simulink model "ec_fixed_config_subsys"  (Simulink 10.0)
settings: Solver=FixedStepDiscrete  StartTime=0.0  StopTime=20  RelTol=1e-3
PreLoadFcn:
  | ec_fixed_setup;
StartFcn:
  | tic;
StopFcn:
  | toc;
undefined symbols (not defined in the file): Fs, pic_frame_size
libraries: dspsrcs4 x9, ec_lib x6, simulink x6
settings Model: Creator=Kerry Schutz  LastModifiedBy=bhisma
settings DataIOCC: LimitDataPoints=on  SignalLoggingSaveFormat=ModelDataLogs
settings OptimizationCC: DefaultParameterBehavior=Inlined  InlineInvariantSignals=on  ExpressionDepthLimit=2147483647  StateBitsets=on  DataBitsets=on  ZeroExternalMemoryAtStartup=off  ZeroInternalMemoryAtStartup=off  EfficientFloat2IntCast=on  LifeSpan=1  EfficientTunableParamExpr=on
settings DebuggingCC: AlgebraicLoopMsg=none  SaveWithParameterizedLinksMsg=none  SolverPrmCheckMsg=warning  FcnCallInpInsideContextMsg=warning  StateNameClashWarn=warning
settings HardwareCC: ProdBitPerInt=16  ProdBitPerPointer=16  ProdBitPerSizeT=16  ProdBitPerPtrDiffT=16  ProdIntDivRoundTo=Zero  ProdEndianess=LittleEndian  ProdWordSize=16  ProdHWDeviceType=Microchip->dsPIC  TargetHWDeviceType=32-bit Generic
settings SFSimCC: SimUseLocalCustomCode=on  SimParseCustomCode=off  MATLABDynamicMemAlloc=off  CustomCodeUndefinedFunction=FilterOut
settings RTWCC: Description=Real-Time Workshop Embedded Coder (no auto configuration)  SystemTargetFile=ert.tlc  GenCodeOnly=on  TemplateMakefile=ert_default_tmf  RTWUseLocalCustomCode=on  CreateSILPILBlock=SIL
settings CodeAppCC: IgnoreCustomStorageClasses=off  CustomSymbolStrType=$N$R$M  InternalIdentifier=Classic  InlinedPrmAccess=Macros
settings ERTTargetCC: TargetFcnLib=ansi_tfl_tmw.mat  GenerateSampleERTMain=on  IncludeMdlTerminateFcn=off  SupportAbsoluteTime=off  PurelyIntegerCode=on  SupportNonFinite=off  SupportComplex=off  InlinedParameterPlacement=NonHierarchical  ERTCustomFileTemplate=example_file_process.tlc  ConvertIfToSwitch=off  SuppressUnreachableDefaultCases=off

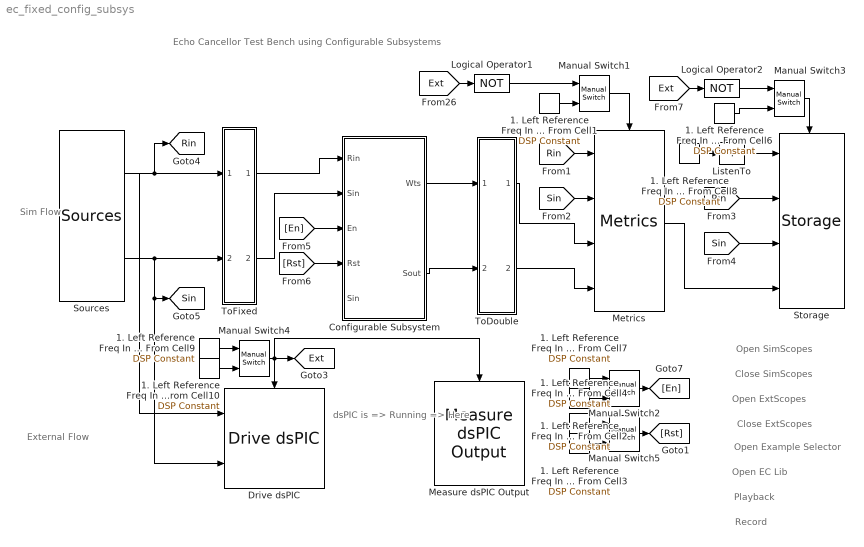
== system ec_fixed_config_subsys ==
  note: Echo Cancellor Test Bench using Configurable Subsystems
  note: Sim
      | Flow
  note: dsPIC is
      | => Running  =>
      |   Here
  note: External
      | Flow
  note: Playback
  note: Record
  note: Open EC Lib
  note: Open Example Selector
  note: Close SimScopes
  note: Open ExtScopes
  note: Close ExtScopes
  note: Open SimScopes
  1. Left Reference Freq In Hz From Cell1 : dspsrcs4/DSP Constant  SystemSampleTime=-1  Value=0  SampleMode=Discrete  discreteOutput=Sample-based  continuousOutput=Sample-based  sampTime=pic_frame_size/Fs  framePeriod=pic_frame_size/Fs  dataType=double  isSigned=on  wordLen=16  udDataType=sfix(16)  fracBitsMode=Best precision  numFracBits=15  InterpretAs1D=-inf  Ts=-inf  FramebasedOutput=-inf
      settings: SourceProductName=DSP System Toolbox  SourceProductBaseCode=DS  additionalParams=on
  1. Left Reference Freq In Hz From Cell10 : dspsrcs4/DSP Constant  SystemSampleTime=-1  Value=0  SampleMode=Discrete  discreteOutput=Sample-based  continuousOutput=Sample-based  sampTime=pic_frame_size/Fs  framePeriod=pic_frame_size/Fs  dataType=double  isSigned=on  wordLen=16  udDataType=sfix(16)  fracBitsMode=Best precision  numFracBits=15  InterpretAs1D=-inf  Ts=-inf  FramebasedOutput=-inf
      settings: SourceProductName=DSP System Toolbox  SourceProductBaseCode=DS  additionalParams=on
  1. Left Reference Freq In Hz From Cell2 : dspsrcs4/DSP Constant  SystemSampleTime=-1  Value=0  SampleMode=Discrete  discreteOutput=Sample-based  continuousOutput=Sample-based  sampTime=pic_frame_size/Fs  framePeriod=pic_frame_size/Fs  dataType=int16  isSigned=on  wordLen=16  udDataType=sfix(16)  fracBitsMode=Best precision  numFracBits=15  InterpretAs1D=-inf  Ts=-inf  FramebasedOutput=-inf
      settings: SourceProductName=DSP System Toolbox  SourceProductBaseCode=DS  additionalParams=on
  1. Left Reference Freq In Hz From Cell3 : dspsrcs4/DSP Constant  SystemSampleTime=-1  Value=0  SampleMode=Discrete  discreteOutput=Sample-based  continuousOutput=Sample-based  sampTime=pic_frame_size/Fs  framePeriod=pic_frame_size/Fs  dataType=int16  isSigned=on  wordLen=16  udDataType=sfix(16)  fracBitsMode=Best precision  numFracBits=15  InterpretAs1D=-inf  Ts=-inf  FramebasedOutput=-inf
      settings: SourceProductName=DSP System Toolbox  SourceProductBaseCode=DS  additionalParams=on
  1. Left Reference Freq In Hz From Cell4 : dspsrcs4/DSP Constant  SystemSampleTime=-1  Value=1  SampleMode=Discrete  discreteOutput=Sample-based  continuousOutput=Sample-based  sampTime=pic_frame_size/Fs  framePeriod=pic_frame_size/Fs  dataType=int16  isSigned=on  wordLen=16  udDataType=sfix(16)  fracBitsMode=Best precision  numFracBits=15  InterpretAs1D=-inf  Ts=-inf  FramebasedOutput=-inf
      settings: SourceProductName=DSP System Toolbox  SourceProductBaseCode=DS  additionalParams=on
  1. Left Reference Freq In Hz From Cell6 : dspsrcs4/DSP Constant  SystemSampleTime=-1  Value=0  SampleMode=Discrete  discreteOutput=Sample-based  continuousOutput=Sample-based  sampTime=pic_frame_size/Fs  framePeriod=2  dataType=double  isSigned=on  wordLen=16  udDataType=sfix(16)  fracBitsMode=Best precision  numFracBits=15  InterpretAs1D=-inf  Ts=-inf  FramebasedOutput=-inf
      settings: SourceProductName=DSP System Toolbox  SourceProductBaseCode=DS  additionalParams=on
  1. Left Reference Freq In Hz From Cell7 : dspsrcs4/DSP Constant  SystemSampleTime=-1  Value=1  SampleMode=Discrete  discreteOutput=Sample-based  continuousOutput=Sample-based  sampTime=pic_frame_size/Fs  framePeriod=pic_frame_size/Fs  dataType=int16  isSigned=on  wordLen=16  udDataType=sfix(16)  fracBitsMode=Best precision  numFracBits=15  InterpretAs1D=-inf  Ts=-inf  FramebasedOutput=-inf
      settings: SourceProductName=DSP System Toolbox  SourceProductBaseCode=DS  additionalParams=on
  1. Left Reference Freq In Hz From Cell8 : dspsrcs4/DSP Constant  SystemSampleTime=-1  Value=1  SampleMode=Discrete  discreteOutput=Sample-based  continuousOutput=Sample-based  sampTime=pic_frame_size/Fs  framePeriod=2  dataType=double  isSigned=on  wordLen=16  udDataType=sfix(16)  fracBitsMode=Best precision  numFracBits=15  InterpretAs1D=-inf  Ts=-inf  FramebasedOutput=-inf
      settings: SourceProductName=DSP System Toolbox  SourceProductBaseCode=DS  additionalParams=on
  1. Left Reference Freq In Hz From Cell9 : dspsrcs4/DSP Constant  SystemSampleTime=-1  Value=1  SampleMode=Discrete  discreteOutput=Sample-based  continuousOutput=Sample-based  sampTime=pic_frame_size/Fs  framePeriod=pic_frame_size/Fs  dataType=double  isSigned=on  wordLen=16  udDataType=sfix(16)  fracBitsMode=Best precision  numFracBits=15  InterpretAs1D=-inf  Ts=-inf  FramebasedOutput=-inf
      settings: SourceProductName=DSP System Toolbox  SourceProductBaseCode=DS  additionalParams=on
  Configurable Subsystem : Subsystem  BlockChoice=SLM16 codegen
      settings: AttributesFormatString=%<BlockChoice>  MemberBlocks=LCT sim,SLM16 codegen,SLM16 sim,SLP FORi,SLP Force
      settings: TemplateBlock=|
      | ec_lib/Configurable
      | Subsystem
  Drive dsPIC : ec_lib/Drive dsPIC  SystemSampleTime=-1
  ListenTo : simulink/Math Operations/Slider Gain  SystemSampleTime=-1  low=0  gain=4  high=10
  Logical Operator1 : Logic  Operator=NOT  AllPortsSameDT=off  OutDataTypeStr=boolean
  Logical Operator2 : Logic  Operator=NOT  AllPortsSameDT=off  OutDataTypeStr=boolean
  Manual Switch1 : simulink/Signal Routing/Manual Switch  SystemSampleTime=-1  sw=1  action=0  varsize=off
      settings: SourceProductName=Simulink  SourceProductBaseCode=SL
  Manual Switch2 : simulink/Signal Routing/Manual Switch  SystemSampleTime=-1  sw=1  action=0  varsize=off
      settings: SourceProductName=Simulink  SourceProductBaseCode=SL
  Manual Switch3 : simulink/Signal Routing/Manual Switch  SystemSampleTime=-1  sw=1  action=0  varsize=off
      settings: SourceProductName=Simulink  SourceProductBaseCode=SL
  Manual Switch4 : simulink/Signal Routing/Manual Switch  SystemSampleTime=-1  sw=0  action=0  varsize=off
      settings: SourceProductName=Simulink  SourceProductBaseCode=SL
  Manual Switch5 : simulink/Signal Routing/Manual Switch  SystemSampleTime=-1  sw=0  action=0  varsize=off
      settings: SourceProductName=Simulink  SourceProductBaseCode=SL
  Measure dsPIC Output : ec_lib/Measure dsPIC Output  SystemSampleTime=-1
  Metrics : ec_lib/Metrics  SystemSampleTime=-1
  Sources : ec_lib/Sources  SystemSampleTime=-1
  Storage : ec_lib/Storage  SystemSampleTime=-1
  ToDouble : Subsystem
  ToFixed : Subsystem
  tag scope: Ext=global, Rin=global, Sin=global
  wires:
  1. Left Reference Freq In Hz From Cell6/1 -> Manual Switch3/2
  Manual Switch3/1 -> Storage/Enable
  1. Left Reference Freq In Hz From Cell10/1 -> Manual Switch4/2
  1. Left Reference Freq In Hz From Cell9/1 -> Manual Switch4/1
  Manual Switch4/1 -> [Ext], Drive dsPIC/Enable, Measure dsPIC Output/Enable
  ListenTo/1 -> Storage/1
  1. Left Reference Freq In Hz From Cell8/1 -> ListenTo/1
  ToFixed/1(Rin) -> Configurable Subsystem/1(Rin)
  Configurable Subsystem/1(Wts) -> ToDouble/1(In1)
  Configurable Subsystem/2(Sout) -> ToDouble/2(In2)
  Sources/2 -> ToFixed/2(" In2"), [Sin], Drive dsPIC/2
  Sources/1 -> ToFixed/1(In1), [Rin], Drive dsPIC/1
  ToDouble/1(Wts) -> Metrics/3
  ToDouble/2(Sout) -> Metrics/4
  Metrics/1 -> Storage/4
  1. Left Reference Freq In Hz From Cell1/1 -> Manual Switch1/2
  Manual Switch1/1 -> Metrics/Enable
  [Ext] -> Logical Operator1/1
  [Rin] -> Metrics/1
  [Sin] -> Metrics/2
  [Rin] -> Storage/2
  [Sin] -> Storage/3
  1. Left Reference Freq In Hz From Cell7/1 -> Manual Switch2/1
  Manual Switch2/1 -> [En]
  1. Left Reference Freq In Hz From Cell2/1 -> Manual Switch2/2
  1. Left Reference Freq In Hz From Cell4/1 -> Manual Switch5/1
  Manual Switch5/1 -> [Rst]
  1. Left Reference Freq In Hz From Cell3/1 -> Manual Switch5/2
  [En] -> Configurable Subsystem/3(En)
  [Rst] -> Configurable Subsystem/4(Rst)
  Logical Operator1/1 -> Manual Switch1/1
  [Ext] -> Logical Operator2/1
  Logical Operator2/1 -> Manual Switch3/1
  ToFixed/2(Sin) -> Configurable Subsystem/2("Sin ")

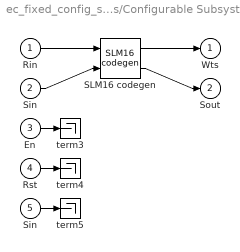
== system ec_fixed_config_subsys/Configurable Subsystem ==
  Rin : Inport
  "Sin " : Inport  Port=2
  En : Inport  Port=3
  Rst : Inport  Port=4
  Sin : Inport  Port=5
  SLM16 codegen : ec_lib/SLM16 codegen  SystemSampleTime=-1
  term3 : Terminator
  term4 : Terminator
  term5 : Terminator
  Wts : Outport
  Sout : Outport  Port=2
  wires:
  Rin/1 -> SLM16 codegen/1
  "Sin "/1 -> SLM16 codegen/2
  SLM16 codegen/1 -> Wts/1
  SLM16 codegen/2 -> Sout/1
  En/1 -> term3/1
  Rst/1 -> term4/1
  Sin/1 -> term5/1

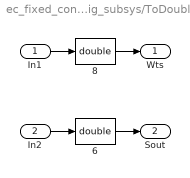
== system ec_fixed_config_subsys/ToDouble ==
  In1 : Inport
  In2 : Inport  Port=2
  " 6" : DataTypeConversion  OutDataTypeStr=double
  " 8" : DataTypeConversion  OutDataTypeStr=double
  Wts : Outport
  Sout : Outport  Port=2
  wires:
  In1/1 -> " 8"/1
  " 8"/1 -> Wts/1
  In2/1 -> " 6"/1
  " 6"/1 -> Sout/1

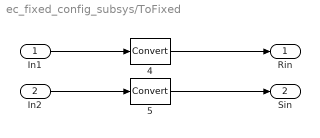
== system ec_fixed_config_subsys/ToFixed ==
  In1 : Inport
  " In2" : Inport  Port=2
  " 4" : DataTypeConversion
  " 5" : DataTypeConversion
  Rin : Outport
  Sin : Outport  Port=2
  wires:
  In1/1 -> " 4"/1
  " 4"/1 -> Rin/1
  " In2"/1 -> " 5"/1
  " 5"/1 -> Sin/1
